simulink subsystem "qrdecomp"  (R2022b)
settings: Solver=VariableStepAuto  StartTime=0.0  StopTime=10.0  RelTol=1e-3
libraries: matrix_library x3, dspsolvers x1
settings Model: Creator=abhij  LastModifiedBy=abhij

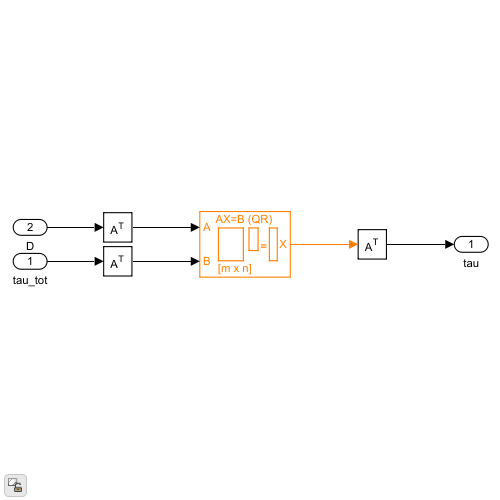
[thumbnail: Simulink's stored preview of the top-level diagram]
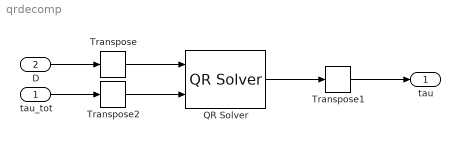
== system qrdecomp ==
  tau_tot : Inport
  D : Inport  Port=2
  QR Solver : dspsolvers/QR Solver  SimulateUsing=Interpreted execution
  Transpose : matrix_library/Transpose
  Transpose1 : matrix_library/Transpose
  Transpose2 : matrix_library/Transpose
  tau : Outport
  wires:
  Transpose1/1 -> tau/1
  Transpose2/1 -> QR Solver/2
  D/1 -> Transpose/1
  tau_tot/1 -> Transpose2/1
  QR Solver/1 -> Transpose1/1
  Transpose/1 -> QR Solver/1
